simulink model "ProjetoRosely"  (Simulink 7.4)
settings: Solver=ode45  StartTime=0.0  StopTime=400  RelTol=1e-3
values from neighbouring files (symbols this model uses):
  B = 0.0078    [trabalhoautomacao_TP1.m]
  J = 3.79    [trabalhoautomacao_TP1.m]
  k3 = 12.8    [trabalhoautomacao_TP1.m]
  kb = 1.28    [trabalhoautomacao_TP1.m]
  La = 1.043    [trabalhoautomacao_TP1.m]
  Ra = 2.4    [trabalhoautomacao_TP1.m]
libraries: simulink x1
settings Model: Creator=Fabiano  LastModifiedBy=Fabiano

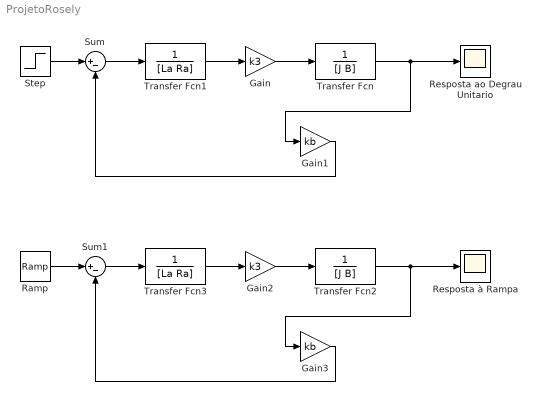
== system ProjetoRosely ==
  Gain : Gain  Gain=k3  ParameterDataType=fixdt(1, 16)  ParameterScaling=2^0  OutDataType=fixdt(1, 16)  OutScaling=2^0
  Gain1 : Gain  Gain=kb  ParameterDataType=fixdt(1, 16)  ParameterScaling=2^0  OutDataType=fixdt(1, 16)  OutScaling=2^0
  Gain2 : Gain  Gain=k3  ParameterDataType=fixdt(1, 16)  ParameterScaling=2^0  OutDataType=fixdt(1, 16)  OutScaling=2^0
  Gain3 : Gain  Gain=kb  ParameterDataType=fixdt(1, 16)  ParameterScaling=2^0  OutDataType=fixdt(1, 16)  OutScaling=2^0
  Ramp : simulink/Sources/Ramp  SystemSampleTime=-1  slope=1  start=0  X0=0
  Resposta ao Degrau Unitario : Scope
      settings: SaveName=ScopeData2
  Resposta à Rampa : Scope
  Step : Step  After=220  SampleTime=0
  Sum : Sum  Inputs=|+-  OutDataType=fixdt(1, 16)  OutScaling=2^0
  Sum1 : Sum  Inputs=|+-  OutDataType=fixdt(1, 16)  OutScaling=2^0
  Transfer Fcn : TransferFcn  Denominator=[J B]
  Transfer Fcn1 : TransferFcn  Denominator=[La Ra]
  Transfer Fcn2 : TransferFcn  Denominator=[J B]
  Transfer Fcn3 : TransferFcn  Denominator=[La Ra]
  wires:
  Sum/1 -> Transfer Fcn1/1
  Transfer Fcn1/1 -> Gain/1
  Gain/1 -> Transfer Fcn/1
  Transfer Fcn/1 -> Gain1/1, Resposta ao Degrau Unitario/1
  Gain1/1 -> Sum/2
  Step/1 -> Sum/1
  Sum1/1 -> Transfer Fcn3/1
  Transfer Fcn3/1 -> Gain2/1
  Gain2/1 -> Transfer Fcn2/1
  Transfer Fcn2/1 -> Gain3/1, Resposta à Rampa/1
  Gain3/1 -> Sum1/2
  Ramp/1 -> Sum1/1
